simulink model "FFUog"  (R2017a)
settings: Solver=ode113  StartTime=0.0  StopTime=10.0  RelTol=1e-6
values from neighbouring files (symbols this model uses):
  param = evalin('base','param')    [getSaveInfo.m]    (also in loadBackUp.m)
settings Model: Creator=www  LastModifiedBy=www
settings SolverCC: MaxConsecutiveMinStep=1000  AlgebraicLoopSolver=LineSearch
settings DataIOCC: SaveOutput=off  SignalLogging=off  DSMLogging=off  SaveTime=off

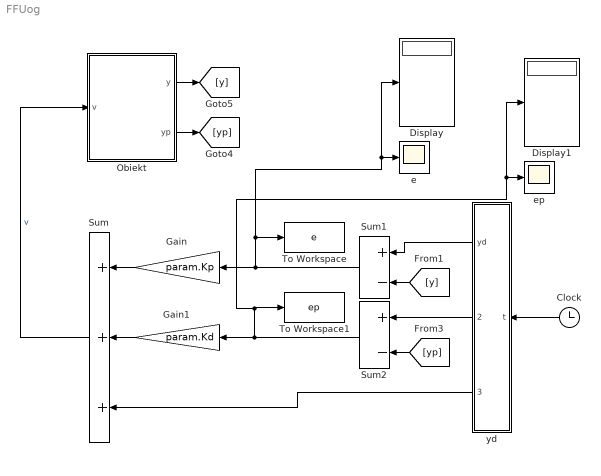
== system FFUog ==
  Clock : Clock
  Display : Display
  Display1 : Display
  Gain : Gain  Gain=param.Kp
  Gain1 : Gain  Gain=param.Kd
  Obiekt : Subsystem
  Sum : Sum  Inputs=+++
  Sum1 : Sum  Inputs=+-
  Sum2 : Sum  Inputs=+-
  To Workspace : ToWorkspace  VariableName=e  SaveFormat=Timeseries  SampleTime=-1
  To Workspace1 : ToWorkspace  VariableName=ep  SaveFormat=Timeseries  SampleTime=-1
  e : Scope
  ep : Scope
  yd : MATLAB Function  TreatAsAtomicUnit=on
  wires:
  Gain/1 -> Sum/1
  Obiekt/2(yp) -> [yp]
  Obiekt/1(y) -> [y]
  yd/2(ydp) -> Sum2/1
  [yp] -> Sum2/2
  [y] -> Sum1/2
  yd/1(yd) -> Sum1/1
  yd/3(ydpp) -> Sum/3
  Sum/1 -> Obiekt/1(v)  "v"
  Clock/1 -> yd/1(t)
  Sum1/1 -> Display/1, e/1, To Workspace/1, Gain/1
  Sum2/1 -> Display1/1, ep/1, To Workspace1/1, Gain1/1
  Gain1/1 -> Sum/2

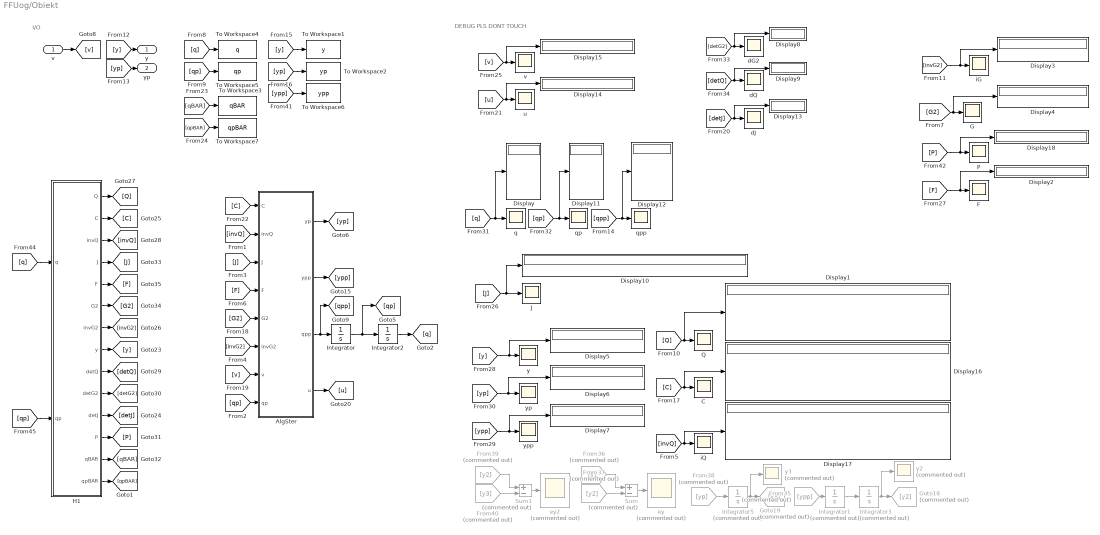
== system FFUog/Obiekt ==
  note: I/O
  note: DEBUG PLS DONT TOUCH
  v : Inport
  AlgSter : MATLAB Function  TreatAsAtomicUnit=on
  C : Scope
  Display{,1..18} (19 alike) : Display
  F : Scope
  From35 : From  Commented=on  GotoTag=ypp
  From36 : From  Commented=on  GotoTag=y
  From37 : From  Commented=on  GotoTag=y2
  From38 : From  Commented=on  GotoTag=yp
  From39 : From  Commented=on  GotoTag=y2
  From40 : From  Commented=on  GotoTag=y3
  G : Scope
  Goto18 : Goto  Commented=on  GotoTag=y2
  Goto19 : Goto  Commented=on  GotoTag=y3
  H1 : MATLAB Function  TreatAsAtomicUnit=on
  Integrator : Integrator  InitialCondition=param.initCond.qp0
  Integrator1 : Integrator  Commented=on  InitialCondition=param.initCond.Yp0
  Integrator2 : Integrator  InitialCondition=param.initCond.q0
  Integrator3 : Integrator  Commented=on  InitialCondition=param.initCond.Y0
  Integrator5 : Integrator  Commented=on  InitialCondition=param.initCond.Y0
  J : Scope
  P : Scope
  Q : Scope
  Sum : Sum  Commented=on  Inputs=+-
  Sum1 : Sum  Commented=on  Inputs=+-
  To Workspace1 : ToWorkspace  VariableName=y  SaveFormat=Timeseries  SampleTime=-1
  To Workspace2 : ToWorkspace  VariableName=yp  SaveFormat=Timeseries  SampleTime=-1
  To Workspace3 : ToWorkspace  VariableName=qBAR  SaveFormat=Timeseries  SampleTime=-1
  To Workspace4 : ToWorkspace  VariableName=q  SaveFormat=Timeseries  SampleTime=-1
  To Workspace5 : ToWorkspace  VariableName=qp  SaveFormat=Timeseries  SampleTime=-1
  To Workspace6 : ToWorkspace  VariableName=ypp  SaveFormat=Timeseries  SampleTime=-1
  To Workspace7 : ToWorkspace  VariableName=qpBAR  SaveFormat=Timeseries  SampleTime=-1
  dG2 : Scope
  dJ : Scope
  dQ : Scope
  ey : Scope  Commented=on
  ey2 : Scope  Commented=on
  iG : Scope
  iQ : Scope
  q : Scope
  qp : Scope
  qpp : Scope
  "u  " : Scope
  "v  " : Scope
  "y " : Scope
  y2 : Scope  Commented=on
  y3 : Scope  Commented=on
  "yp " : Scope
  ypp : Scope
  y : Outport
  yp : Outport  Port=2
  wires:
  v/1 -> [v]
  [G2] -> AlgSter/5(G2)
  [J] -> AlgSter/3(J)
  [v] -> AlgSter/7(v)
  [q] -> To Workspace4/1
  [yp] -> yp/1
  [yp] -> To Workspace2/1
  [y] -> To Workspace1/1
  AlgSter/2(ypp) -> [ypp]
  [y] -> y/1
  [qp] -> To Workspace5/1
  AlgSter/1(yp) -> [yp]
  [F] -> AlgSter/4(F)
  [C] -> AlgSter/1(C)
  [invQ] -> AlgSter/2(invQ)
  [qp] -> AlgSter/8(qp)
  [Q] -> Display1/1, Q/1
  [C] -> Display16/1, C/1
  [invQ] -> Display17/1, iQ/1
  [J] -> Display10/1, J/1
  [y] -> Display5/1, "y "/1
  [yp] -> Display6/1, "yp "/1
  [ypp] -> Display7/1, ypp/1
  [q] -> Display/1, q/1
  [qp] -> qp/1, Display11/1
  [detG2] -> Display8/1, dG2/1
  [detQ] -> Display9/1, dQ/1
  Integrator1/1 -> Integrator3/1
  From35/1 -> Integrator1/1
  Integrator3/1 -> y2/1, Goto18/1
  From36/1 -> Sum/1
  From37/1 -> Sum/2
  Sum/1 -> ey/1
  From38/1 -> Integrator5/1
  Integrator5/1 -> y3/1, Goto19/1
  From40/1 -> Sum1/2
  From39/1 -> Sum1/1
  Sum1/1 -> ey2/1
  [ypp] -> To Workspace6/1
  [F] -> Display2/1, F/1
  AlgSter/3(qpp) -> [qpp], Integrator/1
  Integrator/1 -> [qp], Integrator2/1
  Integrator2/1 -> [q]
  [invG2] -> AlgSter/6(invG2)
  [invG2] -> Display3/1, iG/1
  [G2] -> Display4/1, G/1
  [qpp] -> Display12/1, qpp/1
  [detJ] -> Display13/1, dJ/1
  [u] -> Display14/1, "u  "/1
  [v] -> Display15/1, "v  "/1
  AlgSter/4(u) -> [u]
  [P] -> Display18/1, P/1
  H1/14(qpBAR) -> [qpBAR]
  H1/8(y) -> [y]
  H1/11(detJ) -> [detJ]
  H1/5(F) -> [F]
  H1/3(invQ) -> [invQ]
  H1/2(C) -> [C]
  H1/10(detG2) -> [detG2]
  H1/4(J) -> [J]
  [qp] -> H1/2(qp)
  H1/7(invG2) -> [invG2]
  H1/6(G2) -> [G2]
  H1/9(detQ) -> [detQ]
  H1/1(Q) -> [Q]
  [q] -> H1/1(q)
  H1/12(P) -> [P]
  H1/13(qBAR) -> [qBAR]
  [qBAR] -> To Workspace3/1
  [qpBAR] -> To Workspace7/1

== matlab function FFUog/Obiekt/H1 ==
  data: Q output; C output; q input; qp input; invQ output; J output; F output; G2 output; invG2 output; y output; detQ output; detG2 output; detJ output; P output; qBAR output; qpBAR output
function [Q,C,invQ,J,F,G2,invG2,y,detQ,detG2,detJ,P,qBAR,qpBAR] = fcn(q,qp)

y=[q(1)+2.*cos(q(4)+q(3))+cos(q(4)+q(5)+q(3)),q(2)+2.*sin(q(4)+q(3))+sin(q(4)+q(5)+q(3))];
J=[1,0,(-2).*sin(q(4)+q(3))+(-1).*sin(q(4)+q(5)+q(3)),(-2).*sin(q(4)+q(3))+(-1).*sin( ...
  q(4)+q(5)+q(3)),(-1).*sin(q(4)+q(5)+q(3));0,1,2.*cos(q(4)+q(3))+cos(q(4)+q(5)+q(3)),2.*cos( ...
  q(4)+q(3))+cos(q(4)+q(5)+q(3)),cos(q(4)+q(5)+q(3))];
F=[3.*((-397649)+117045.*cos(2.*q(5))).^(-1).*((-7123).*(qp(3)+qp(4)).^2.* ...
  cos(q(4)+q(3))+3.*((-4335).*(qp(3)+qp(4)+qp(5)).^2.*cos(q(4)+(-1).*q(5)+q(3))+ ...
  31711.*(qp(3)+qp(4)+qp(5)).^2.*cos(q(4)+q(5)+q(3))+41157.*(qp(3)+qp(4)).^2.*cos(q(4)+ ...
  2.*q(5)+q(3))));3.*((-397649)+117045.*cos(2.*q(5))).^(-1).*((-7123).*( ...
  qp(3)+qp(4)).^2.*sin(q(4)+q(3))+3.*((-4335).*(qp(3)+qp(4)+qp(5)).^2.*sin(q(4)+(-1) ...
  .*q(5)+q(3))+31711.*(qp(3)+qp(4)+qp(5)).^2.*sin(q(4)+q(5)+q(3))+41157.*(qp(3)+qp(4)) ...
  .^2.*sin(q(4)+2.*q(5)+q(3))))];
G2=[306.*((-397649)+117045.*cos(2.*q(5))).^(-1).*(13.*sin(q(4)+q(3))+(-54).* ...
  sin(q(4)+2.*q(5)+q(3))),9.*((-1988245)+585225.*cos(2.*q(5))).^(-1).*(( ...
  -2210).*sin(q(4)+q(3))+(-13005).*sin(q(4)+(-1).*q(5)+q(3))+79179.*sin(q(4)+q(5)+q(3)) ...
  +9180.*sin(q(4)+2.*q(5)+q(3)));306.*((-397649)+117045.*cos(2.*q(5))).^(-1) ...
  .*((-13).*cos(q(4)+q(3))+54.*cos(q(4)+2.*q(5)+q(3))),9.*((-1988245)+585225.* ...
  cos(2.*q(5))).^(-1).*(2210.*cos(q(4)+q(3))+13005.*cos(q(4)+(-1).*q(5)+q(3))+( ...
  -79179).*cos(q(4)+q(5)+q(3))+(-9180).*cos(q(4)+2.*q(5)+q(3)))];
invG2=[(1/3672).*((-2210).*cos(q(4)+q(3))+(-13005).*cos(q(4)+(-1).*q(5)+q(3))+ ...
  79179.*cos(q(4)+q(5)+q(3))+9180.*cos(q(4)+2.*q(5)+q(3))).*csc(q(5)),(1/3672).*csc( ...
  q(5)).*((-2210).*sin(q(4)+q(3))+(-13005).*sin(q(4)+(-1).*q(5)+q(3))+79179.*sin( ...
  q(4)+q(5)+q(3))+9180.*sin(q(4)+2.*q(5)+q(3)));(5/108).*((-13).*cos(q(4)+q(3))+54.* ...
  cos(q(4)+2.*q(5)+q(3))).*csc(q(5)),(5/108).*csc(q(5)).*((-13).*sin(q(4)+q(3))+54.* ...
  sin(q(4)+2.*q(5)+q(3)))];
P=[(-2).*(qp(3)+qp(4)).^2.*cos(q(4)+q(3))+(-1).*(qp(3)+qp(4)+qp(5)).^2.*cos(q(4)+q(5)+ ...
  q(3));(-2).*(qp(3)+qp(4)).^2.*sin(q(4)+q(3))+(-1).*(qp(3)+qp(4)+qp(5)).^2.*sin(q(4)+ ...
  q(5)+q(3))];
Q=[41,0,(-31).*sin(q(4)+q(3))+(-5).*sin(q(4)+q(5)+q(3)),(-31).*sin(q(4)+q(3))+(-5).* ...
  sin(q(4)+q(5)+q(3)),(-5).*sin(q(4)+q(5)+q(3));0,41,31.*cos(q(4)+q(3))+5.*cos(q(4)+q(5)+q(3)) ...
  ,31.*cos(q(4)+q(3))+5.*cos(q(4)+q(5)+q(3)),5.*cos(q(4)+q(5)+q(3));(-31).*sin(q(4)+q(3))+( ...
  -5).*sin(q(4)+q(5)+q(3)),31.*cos(q(4)+q(3))+5.*cos(q(4)+q(5)+q(3)),68+20.*cos(q(5)),58+ ...
  20.*cos(q(5)),(5/3).*(2+6.*cos(q(5)));(-31).*sin(q(4)+q(3))+(-5).*sin(q(4)+ ...
  q(5)+q(3)),31.*cos(q(4)+q(3))+5.*cos(q(4)+q(5)+q(3)),58+20.*cos(q(5)),58+20.*cos(q(5)), ...
  (5/3).*(2+6.*cos(q(5)));(-5).*sin(q(4)+q(5)+q(3)),5.*cos(q(4)+q(5)+q(3)),(5/3).*( ...
  2+6.*cos(q(5))),(5/3).*(2+6.*cos(q(5))),(10/3)];
C=[0,0,(1/2).*((-62).*(qp(3)+qp(4)).*cos(q(4)+q(3))+(-10).*(qp(3)+qp(4)+qp(5)).* ...
  cos(q(4)+q(5)+q(3))),(1/2).*((-62).*(qp(3)+qp(4)).*cos(q(4)+q(3))+(-10).*(qp(3)+qp(4)+ ...
  qp(5)).*cos(q(4)+q(5)+q(3))),(-5).*(qp(3)+qp(4)+qp(5)).*cos(q(4)+q(5)+q(3));0,0,(1/2).*( ...
  (-62).*(qp(3)+qp(4)).*sin(q(4)+q(3))+(-10).*(qp(3)+qp(4)+qp(5)).*sin(q(4)+q(5)+q(3))),( ...
  1/2).*((-62).*(qp(3)+qp(4)).*sin(q(4)+q(3))+(-10).*(qp(3)+qp(4)+qp(5)).*sin(q(4)+ ...
  q(5)+q(3))),(-5).*(qp(3)+qp(4)+qp(5)).*sin(q(4)+q(5)+q(3));0,0,(-10).*qp(5).*sin(q(5)),( ...
  -10).*qp(5).*sin(q(5)),(-10).*(qp(3)+qp(4)+qp(5)).*sin(q(5));0,0,(-10).*qp(5).* ...
  sin(q(5)),(-10).*qp(5).*sin(q(5)),(-10).*(qp(3)+qp(4)+qp(5)).*sin(q(5));0,0,10.* ...
  (qp(3)+qp(4)).*sin(q(5)),10.*(qp(3)+qp(4)).*sin(q(5)),0];
invQ=[2.*((-397649)+117045.*cos(2.*q(5))).^(-1).*(2295.*cos(2.*q(5))+1488.* ...
  cos(2.*(q(4)+q(3)))+(-55).*(128+3.*cos(2.*(q(4)+q(5)+q(3))))),6.*((-397649)+ ...
  117045.*cos(2.*q(5))).^(-1).*(496.*sin(2.*(q(4)+q(3)))+(-55).*sin(2.*(q(4)+ ...
  q(5)+q(3)))),0,3.*((-397649)+117045.*cos(2.*q(5))).^(-1).*((-3389).*sin( ...
  q(4)+q(3))+765.*sin(q(4)+2.*q(5)+q(3))),3.*((-397649)+117045.*cos(2.*q(5))).^( ...
  -1).*(3389.*sin(q(4)+q(3))+4743.*sin(q(4)+(-1).*q(5)+q(3))+(-2939).*sin(q(4)+q(5)+ ...
  q(3))+(-765).*sin(q(4)+2.*q(5)+q(3)));6.*((-397649)+117045.*cos(2.*q(5))).^( ...
  -1).*(496.*sin(2.*(q(4)+q(3)))+(-55).*sin(2.*(q(4)+q(5)+q(3)))),2.*((-397649)+ ...
  117045.*cos(2.*q(5))).^(-1).*((-7040)+2295.*cos(2.*q(5))+(-1488).*cos( ...
  2.*(q(4)+q(3)))+165.*cos(2.*(q(4)+q(5)+q(3)))),0,3.*((-397649)+117045.*cos(2.* ...
  q(5))).^(-1).*(3389.*cos(q(4)+q(3))+(-765).*cos(q(4)+2.*q(5)+q(3))),3.*(( ...
  -397649)+117045.*cos(2.*q(5))).^(-1).*((-3389).*cos(q(4)+q(3))+(-4743).* ...
  cos(q(4)+(-1).*q(5)+q(3))+2939.*cos(q(4)+q(5)+q(3))+765.*cos(q(4)+2.*q(5)+q(3)));0,0,( ...
  1/10),(-1/10),0;3.*((-397649)+117045.*cos(2.*q(5))).^(-1).*((-3389) ...
  .*sin(q(4)+q(3))+765.*sin(q(4)+2.*q(5)+q(3))),3.*((-397649)+117045.*cos(2.*q(5)) ...
  ).^(-1).*(3389.*cos(q(4)+q(3))+(-765).*cos(q(4)+2.*q(5)+q(3))),(-1/10),(( ...
  -562469)+117045.*cos(2.*q(5))).*((-3976490)+1170450.*cos(2.*q(5))).^( ...
  -1),246.*(67+153.*cos(q(5))).*((-397649)+117045.*cos(2.*q(5))).^(-1); ...
  3.*((-397649)+117045.*cos(2.*q(5))).^(-1).*(3389.*sin(q(4)+q(3))+4743.* ...
  sin(q(4)+(-1).*q(5)+q(3))+(-2939).*sin(q(4)+q(5)+q(3))+(-765).*sin(q(4)+2.*q(5)+q(3))), ...
  3.*((-397649)+117045.*cos(2.*q(5))).^(-1).*((-3389).*cos(q(4)+q(3))+( ...
  -4743).*cos(q(4)+(-1).*q(5)+q(3))+2939.*cos(q(4)+q(5)+q(3))+765.*cos(q(4)+2.*q(5)+q(3)) ...
  ),0,246.*(67+153.*cos(q(5))).*((-397649)+117045.*cos(2.*q(5))).^(-1),( ...
  -4428).*(232+85.*cos(q(5))).*((-1988245)+585225.*cos(2.*q(5))).^(-1)]; ...
  
x1bar=q(1)+(31/41).*cos(q(4)+q(3))+(5/41).*cos(q(4)+q(5)+q(3));
y1bar=q(2)+(31/41).*sin(q(4)+q(3))+(5/41).*sin(q(4)+q(5)+q(3));
xpbar=qp(1)+(-31/41).*(qp(3)+qp(4)).*sin(q(4)+q(3))+(-5/41).*(qp(3)+qp(4)+qp(5)).*sin(q(4)+ ...
  q(5)+q(3));
ypbar=qp(2)+(31/41).*(qp(3)+qp(4)).*cos(q(4)+q(3))+(5/41).*(qp(3)+qp(4)+qp(5)).*cos(q(4)+ ...
  q(5)+q(3));







qBAR=[x1bar;y1bar];
qpBAR=[xpbar;ypbar];

detQ=det(Q);
detJ=1337;
detG2=det(G2);

== matlab function FFUog/Obiekt/AlgSter ==
  data: C input; invQ input; yp output; ypp output; J input; F input; G2 input; invG2 input; v input; qp input; qpp output; u output
function [yp,ypp,qpp,u] = fcn(C,invQ,J,F,G2,invG2,v,qp)

yp=J*qp;
ypp=F+G2*v;

u=invG2*(-F+v);
qpp=invQ*([0;0;0;u]-C*qp);

== matlab function FFUog/yd ==
  data: yd output; ydp output; ydpp output; t input
function [yd,ydp, ydpp] = fcn(t)
% sina=0.2;
% sinb=0.2;
% sinn=sina*sin(sinb*t);
% sinp=sina*sinb*cos(sinb*t);
% sinpp=-sina*sinb^2*sin(sinb*t);
% 
% dln=1;
% lna=0.01;
% lnb=30;
% lndt=1;
% ln=dln+lna*log(lnb*(t+lndt));
% lnp=lna/(t+lndt);
% lnpp=-lna/(t+lndt)^2;
% 
% yd=[sinn;
%     ln];
% ydp=[sinp;
%    lnp];
% ydpp=[sinpp;
%      lnpp];

yd=[t;
    t];
ydp=[1;
   1];
ydpp=[0;
     0];
